simulink subsystem "directFFcontroller"  (R2021a)
settings: Solver=VariableStepAuto  StartTime=0.0  StopTime=10.0  RelTol=1e-3
settings Model: Creator=chukh  LastModifiedBy=20210123

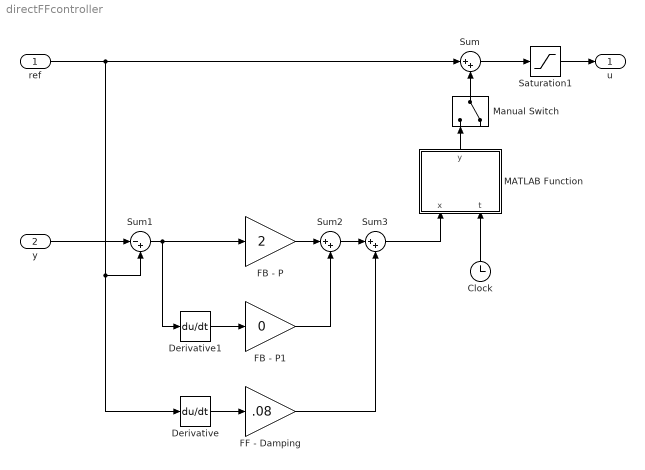
== system directFFcontroller ==
  ref : Inport
  y : Inport  Port=2
  Clock : Clock
  Derivative : Derivative
  Derivative1 : Derivative
  FB - P : Gain  Gain=2
  FB - P1 : Gain  Gain=0
  FF - Damping : Gain  Gain=.08
  MATLAB Function : MATLAB Function  TreatAsAtomicUnit=on
  Manual Switch : ManualSwitch  CurrentSetting=0
  Saturation1 : Saturate  UpperLimit=1  LowerLimit=0
  Sum : Sum  Inputs=|++
  Sum1 : Sum  Inputs=|-+
  Sum2 : Sum  Inputs=|++
  Sum3 : Sum  Inputs=|++
  u : Outport
  wires:
  Saturation1/1 -> u/1
  ref/1 -> Sum/1, Derivative/1, Sum1/2
  FB - P/1 -> Sum2/1
  Manual Switch/1 -> Sum/2
  y/1 -> Sum1/1
  Derivative/1 -> FF - Damping/1
  Sum1/1 -> FB - P/1, Derivative1/1
  Sum2/1 -> Sum3/1
  FB - P1/1 -> Sum2/2
  Derivative1/1 -> FB - P1/1
  Clock/1 -> MATLAB Function/2(t)
  MATLAB Function/1(y) -> Manual Switch/1
  Sum3/1 -> MATLAB Function/1(x)
  FF - Damping/1 -> Sum3/2
  Sum/1 -> Saturation1/1

== matlab function directFFcontroller/MATLAB Function ==
  data: x input; t input; y output
function y = smoothstep(x,t)
y = x*min(.1*t,1);
end
